simulink model "Simulink_Offline_Horizontal_Control_2019"  (R2019b)
settings: Solver=VariableStepAuto  StartTime=0.0  StopTime=10.0  RelTol=1e-3
values from neighbouring files (symbols this model uses):
  C = eye(4)    [Compensator_StartUp.m]
  D = zeros(4,1)    [Compensator_StartUp.m]
  Kd = G.Kd    [Compensator_StartUp.m]
  Ki = G.Ki    [Compensator_StartUp.m]
  Kp = G.Kp    [Compensator_StartUp.m]
  voltage_max = 10    [Compensator_StartUp.m]
undefined symbols (not defined in the file or in its folder): A, B
libraries: cstblocks x4, simulink x2
settings Model: Creator=utente  LastModifiedBy=utente

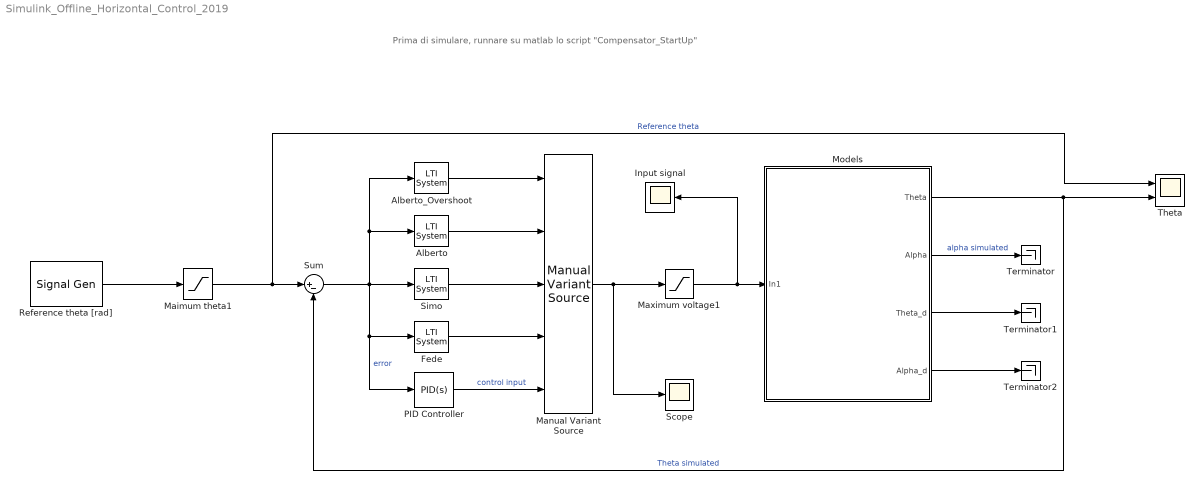
== system Simulink_Offline_Horizontal_Control_2019 ==
  note: Prima di simulare, runnare su matlab lo script "Compensator_StartUp"
  Alberto : cstblocks/LTI System  sys=R2  IC=[]
  Alberto_Overshoot : cstblocks/LTI System  sys=R1  IC=[]
  Fede : cstblocks/LTI System  sys=R4  IC=[]
  Input signal : Scope
  Maimum theta1 : Saturate  UpperLimit=pi/2  LowerLimit=-pi/2
  Manual Variant Source : simulink/Signal Routing/Manual Variant Source  NumChoices=5  LabelModeActiveChoice=V_1
      settings: SourceProductName=Simulink
  Maximum voltage1 : Saturate  UpperLimit=voltage_max  LowerLimit=-voltage_max
  Models : Subsystem
  PID Controller : simulink/Continuous/PID Controller  Controller=PID  Form=Parallel  TimeDomain=Continuous-time  SampleTime=-1  IntegratorMethod=Forward Euler  FilterMethod=Forward Euler  ControllerParametersSource=internal  P=Kp  I=Ki  D=Kd  UseFilter=on  N=10  TunerSelectOption=Transfer Function Based (PID Tuner App)  InitialConditionSource=internal  InitialConditionForIntegrator=0  InitialConditionForFilter=0  DifferentiatorICPrevScaledInput=0  ExternalReset=none  TrackingMode=off  Kt=1  LimitOutput=off  UpperSaturationLimit=inf  LowerSaturationLimit=-inf  LinearizeAsGain=on  AntiWindupMode=none  Kb=1  POutMin=[]  POutMax=[]  IOutMin=[]  IOutMax=[]  DOutMin=[]  DOutMax=[]  NOutMin=[]  NOutMax=[]  SumOutMin=[]  SumOutMax=[]  SaturationOutMin=[]  SaturationOutMax=[]  PParamMin=[]  PParamMax=[]  IParamMin=[]  IParamMax=[]  DParamMin=[]  DParamMax=[]  NParamMin=[]  NParamMax=[]  KbParamMin=[]  KbParamMax=[]  KtParamMin=[]  KtParamMax=[]  KbOutMin=[]  KbOutMax=[]  KtOutMin=[]  KtOutMax=[]  IntegratorOutMin=[]  IntegratorOutMax=[]  FilterOutMin=[]  FilterOutMax=[]  SumI1OutMin=[]  SumI1OutMax=[]  SumI2OutMin=[]  SumI2OutMax=[]  SumI3OutMin=[]  SumI3OutMax=[]  SumI4OutMin=[]  SumI4OutMax=[]  SumDOutMin=[]  SumDOutMax=[]  DifferentiatorOutMin=[]  DifferentiatorOutMax=[]  FilterDiffOutCoefMin=[]  FilterDiffOutCoefMax=[]  ReciprocalOutMin=[]  ReciprocalOutMax=[]  SumDenOutMin=[]  SumDenOutMax=[]  SumNumOutMin=[]  SumNumOutMax=[]  DivideOutMin=[]  DivideOutMax=[]  IntegratorContinuousStateAttributes=''  IntegratorStateMustResolveToSignalObject=off  IntegratorRTWStateStorageClass=Auto  FilterContinuousStateAttributes=''  FilterStateMustResolveToSignalObject=off  FilterRTWStateStorageClass=Auto  ParallelPVariant=InternalParameters  IdealPVariant=Disabled  IVariant=InternalParameters  DVariant=InternalParameters  IntegratorVariant=Continuous  SatVariant=Disabled  AWVariant=Passthrough  PCopyVariant=Disabled  TRVariant=Disabled  FdbkBlocksVariant=Forward  IdealPFdbkVariant=Disabled  SatFdbkVariant=Disabled  DerivativeFilterVariant=ContFilter  NVariant=InternalParameters  NCopyVariant=Disabled  FilterICVariant=InternalICsFilter  IntegratorICVariant=InternalICs  ExternalResetVariant=Disabled  TRSumVariant=Passthrough  SumFdbkVariant=Disabled  SumVariant=Sum_PID
  Reference theta [rad] : SignalGenerator  WaveForm=square  Amplitude=pi/4  Frequency=0.5
  Scope : Scope
  Simo : cstblocks/LTI System  sys=R3  IC=[]
  Sum : Sum  Inputs=|+-
  Terminator : Terminator
  Terminator1 : Terminator
  Terminator2 : Terminator
  Theta : Scope  NumInputPorts=2
  wires:
  Models/1(Theta) -> Theta/2, Sum/2  "Theta simulated"
  Models/2(Alpha) -> Terminator/1  "alpha simulated"
  Models/3(Theta_d) -> Terminator1/1
  Models/4(Alpha_d) -> Terminator2/1
  Reference theta [rad]/1 -> Maimum theta1/1
  Maximum voltage1/1 -> Models/1(In1), Input signal/1
  Sum/1 -> Fede/1, PID Controller/1, Simo/1, Alberto_Overshoot/1, Alberto/1  "error"
  Maimum theta1/1 -> Sum/1, Theta/1  "Reference theta"
  Alberto_Overshoot/1 -> Manual Variant Source/1
  Manual Variant Source/1 -> Scope/1, Maximum voltage1/1
  Alberto/1 -> Manual Variant Source/2
  Simo/1 -> Manual Variant Source/3
  Fede/1 -> Manual Variant Source/4
  PID Controller/1 -> Manual Variant Source/5  "control input"

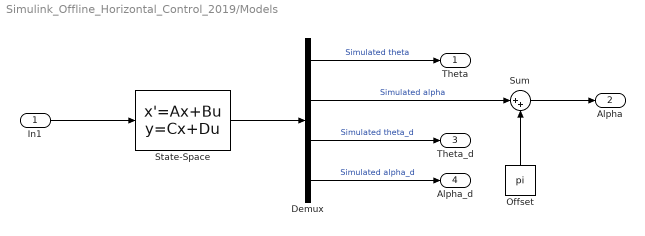
== system Simulink_Offline_Horizontal_Control_2019/Models ==
  In1 : Inport
  Demux : Demux
  Offset : Constant  Value=pi
  State-Space : StateSpace  A=A  B=B  C=C  D=D  InitialCondition=0
  Sum : Sum  Inputs=|++
  Theta : Outport
  Alpha : Outport  Port=2
  Theta_d : Outport  Port=3
  Alpha_d : Outport  Port=4
  wires:
  In1/1 -> State-Space/1
  Demux/1 -> Theta/1  "Simulated theta"
  Demux/2 -> Sum/1  "Simulated alpha"
  State-Space/1 -> Demux/1
  Demux/4 -> Alpha_d/1  "Simulated alpha_d"
  Demux/3 -> Theta_d/1  "Simulated theta_d"
  Sum/1 -> Alpha/1
  Offset/1 -> Sum/2
